simulink model "dcmotor_simulation"  (R2021b)
settings: Solver=VariableStepAuto  StartTime=0.0  StopTime=6  RelTol=1e-3
values from neighbouring files (symbols this model uses):
  La = 0.2    [dcmotor_parameters.m]    (also in simulation.m = 0.1)
  Ra = 1    [dcmotor_parameters.m]    (also in simulation.m = 0.5)
  TL = 0    [dcmotor_parameters.m]    (also in simulation.m = 20)
  Va = 12    [dcmotor_parameters.m]    (also in simulation.m)
undefined symbols (not defined in the file or in its folder): Bm, Jm, Ke
libraries: simulink_extras x2
settings Model: Creator=sacka  LastModifiedBy=sacka

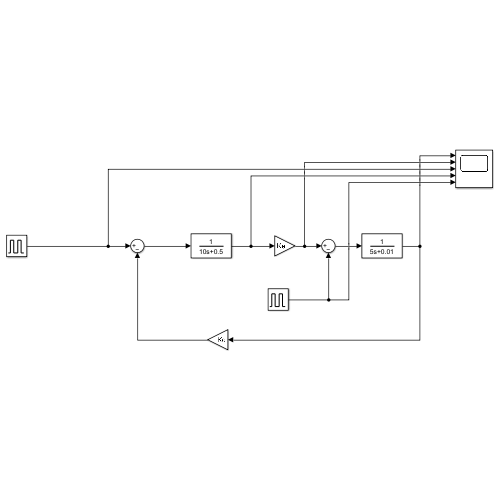
[thumbnail: Simulink's stored preview of the top-level diagram]
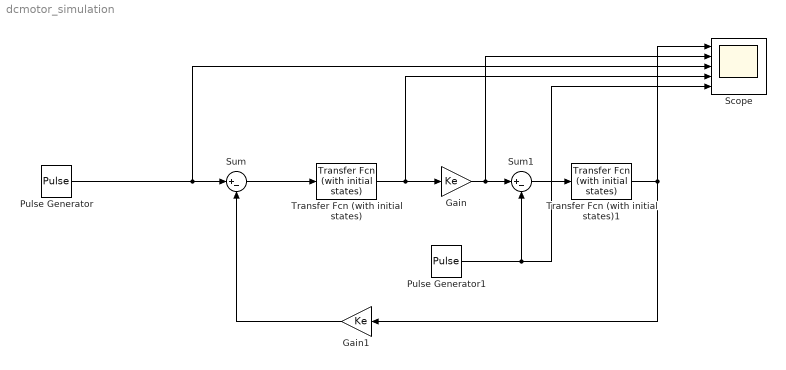
== system dcmotor_simulation ==
  Gain : Gain  Gain=Ke
  Gain1 : Gain  Gain=Ke
  Pulse Generator : DiscretePulseGenerator  PulseType=Time based  Amplitude=Va  Period=30  PulseWidth=90  PhaseDelay=1
  Pulse Generator1 : DiscretePulseGenerator  PulseType=Time based  Amplitude=TL  Period=30  PulseWidth=90  PhaseDelay=6
  Scope : Scope  NumInputPorts=5
  Sum : Sum  Inputs=|+-
  Sum1 : Sum  Inputs=|+-
  Transfer Fcn (with initial states) : simulink_extras/Additional Linear/Transfer Fcn (with initial states)  N=[1]  D=[La Ra]  X0=0
  Transfer Fcn (with initial states)1 : simulink_extras/Additional Linear/Transfer Fcn (with initial states)  N=[1]  D="[Jm  Bm]"  X0=0
  wires:
  Pulse Generator/1 -> Scope/3, Sum/1
  Sum/1 -> Transfer Fcn (with initial states)/1
  Gain/1 -> Scope/2, Sum1/1
  Sum1/1 -> Transfer Fcn (with initial states)1/1
  Transfer Fcn (with initial states)1/1 -> Scope/1, Gain1/1
  Gain1/1 -> Sum/2
  Transfer Fcn (with initial states)/1 -> Scope/4, Gain/1
  Pulse Generator1/1 -> Scope/5, Sum1/2
